simulink model "sowavedec2embd"  (R2012a)
settings: Solver=FixedStepDiscrete  StartTime=0.0  StopTime=inf  RelTol=1e-3
libraries: embdlinuxlib x2
settings Model: ExtModeTrigDuration=100  Creator=harashin  LastModifiedBy=Shogo
settings DataIOCC: LimitDataPoints=on  SaveFormat=Array  ReturnWorkspaceOutputs=off
settings OptimizationCC: ExpressionDepthLimit=2147483647  OptimizeModelRefInitCode=on  LifeSpan=1  SimCompilerOptimization=Off
settings DebuggingCC: UnderspecifiedInitializationDetection=Classic  MergeDetectMultiDrivingBlocksExec=none  FcnCallInpInsideContextMsg=Enable All  FrameProcessingCompatibilityMsg=warning  StateNameClashWarn=warning  StrictBusMsg=Warning  SFUnexpectedBacktrackingDiag=warning  SFNoUnconditionalDefaultTransitionDiag=warning
settings HardwareCC: ProdBitPerPointer=32  ProdLargestAtomicInteger=Long  ProdLargestAtomicFloat=Double  ProdIntDivRoundTo=Undefined  ProdWordSize=32  ProdHWDeviceType=ARM Compatible->ARM Cortex
settings ModelReferenceCC: PropagateSignalLabelsOutOfModel=off
settings SFSimCC: SimUseLocalCustomCode=off
settings RTWCC: SystemTargetFile=realtime.tlc  GenerateMakefile=off  TemplateMakefile=realtime.tmf  Description=Real-Time Toolbox  RTWVerbose=off  ProcessScript=realtime_make_rtw_hook  RTWUseLocalCustomCode=off  RTWCompilerOptimization=Off
settings CodeAppCC: CustomSymbolStrType=$N$R$M
settings STFCustomTargetCC: TargetLibSuffix=.a  CodeReplacementLibrary=ANSI_C  GenerateSampleERTMain=on  ERTCustomFileBanners=on  SupportNonInlinedSFcns=off  SupportVariableSizeSignals=on  GRTInterface=off  SystemTargetFile=realtime.tlc
settings ERTTargetCC: CodeReplacementLibrary=ANSI_C  MultiwordLength=2048  GenerateSampleERTMain=on  ParMdlRefBuildCompliant=off  CompOptLevelCompliant=off  ConcurrentExecutionCompliant=off  CombineOutputUpdateFcns=off  ERTFirstTimeCompliant=off  SupportContinuousTime=on  SupportVariableSizeSignals=on  ModelStepFunctionPrototypeControlCompliant=off  CPPClassGenCompliant=off  ExtModeMexArgs='192.168.111.22' 0 17725  InlinedParameterPlacement=NonHierarchical  ERTSrcFileBannerTemplate=realtime_code_template.cgt  ERTHdrFileBannerTemplate=realtime_code_template.cgt  ERTDataSrcFileTemplate=realtime_code_template.cgt  ERTDataHdrFileTemplate=realtime_code_template.cgt  ERTCustomFileTemplate=realtime_file_process.tlc  ConvertIfToSwitch=off  SuppressUnreachableDefaultCases=off  MemSecPackage=Simulink

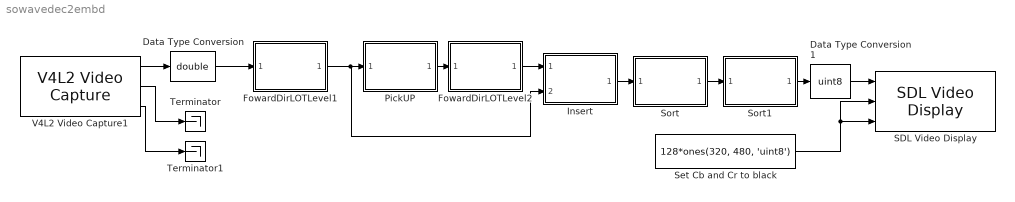
== system sowavedec2embd ==
  Data Type Conversion : DataTypeConversion  OutDataTypeStr=double
  Data Type Conversion1 : DataTypeConversion  OutDataTypeStr=uint8  SaturateOnIntegerOverflow=on
  FowardDirLOTLevel1 : MATLAB Function  TreatAsAtomicUnit=on
      settings: PermitHierarchicalResolution=ParametersOnly
  FowardDirLOTLevel2 : MATLAB Function  TreatAsAtomicUnit=on
      settings: PermitHierarchicalResolution=ParametersOnly
  Insert : MATLAB Function  TreatAsAtomicUnit=on
      settings: PermitHierarchicalResolution=ParametersOnly
  PickUP : MATLAB Function  TreatAsAtomicUnit=on
      settings: PermitHierarchicalResolution=ParametersOnly
  SDL Video Display : embdlinuxlib/SDL Video Display  pixelFormat=YCbCr 4:2:2  pixelOrder=Planar  rowMajor=on  blockPlatform=BeagleBoard
  Set Cb and Cr to black : Constant  Value=128*ones(320, 480, 'uint8')
  Sort : MATLAB Function  TreatAsAtomicUnit=on
      settings: PermitHierarchicalResolution=ParametersOnly
  Sort1 : MATLAB Function  TreatAsAtomicUnit=on
      settings: PermitHierarchicalResolution=ParametersOnly
  Terminator : Terminator
  Terminator1 : Terminator
  V4L2 Video Capture1 : embdlinuxlib/V4L2 Video Capture  m_devName='/dev/video0'  roi=[0, 0, 640, 480]  imSizeSelection=640x480  imSize=[640, 480]  pixelFormat=YCbCr 4:2:2  pixelOrder=Planar  sampleTime=1/10  simOutput=Colorbars  blockPlatform=BeagleBoard
  wires:
  Set Cb and Cr to black/1 -> SDL Video Display/3, SDL Video Display/2
  V4L2 Video Capture1/2 -> Terminator/1
  V4L2 Video Capture1/3 -> Terminator1/1
  V4L2 Video Capture1/1 -> Data Type Conversion/1
  Data Type Conversion1/1 -> SDL Video Display/1
  FowardDirLOTLevel1/1(coefActual) -> Insert/2(srcImg2), PickUP/1(srcImg)
  Data Type Conversion/1 -> FowardDirLOTLevel1/1(srcImg)
  PickUP/1(coefActual) -> FowardDirLOTLevel2/1(srcImg)
  FowardDirLOTLevel2/1(coefActual) -> Insert/1(srcImg1)
  Insert/1(coefActual) -> Sort/1(srcImg)
  Sort/1(coefActual) -> Sort1/1(srcImg)
  Sort1/1(coefActual) -> Data Type Conversion1/1

== matlab function sowavedec2embd/PickUP ==
  data: srcImg input; coefActual output
function coefActual = fcn(srcImg) %#codegen
%[ coefActual ] = coefPickUp(srcImg);
persistent hp;

if isempty(hp)
    
    % Instantiation
    hp = PickUp();
end

% Actual values
coefActual = step(hp,srcImg);

== matlab function sowavedec2embd/FowardDirLOTLevel1 ==
  data: srcImg input; coefActual output
function coefActual = fcn(srcImg) %#codegen 
%[ coefActual ] = forwardDirLot(srcImg);
persistent hf;
if isempty(hf)
    % Instantiation
    hf = ForwardDirLotEmb();
end
% Actual values
coefActual = step(hf,srcImg);

== matlab function sowavedec2embd/FowardDirLOTLevel2 ==
  data: srcImg input; coefActual output
function coefActual = fcn(srcImg) %#codegen
%[ coefActual ] = forwardDirLot(srcImg);
persistent hf;
if isempty(hf)
    % Instantiation
    hf = ForwardDirLotEmb();
end
% Actual values
coefActual = step(hf,srcImg);

== matlab function sowavedec2embd/Insert ==
  data: srcImg1 input; coefActual output; srcImg2 input
function coefActual = fcn(srcImg1,srcImg2) %#codegen
%[ coefActual ] = coefInsert(srcImg1,srcImg2);
persistent hi;

if isempty(hi)
    % Instantiation
    hi = Insert();
end

% Actual values
coefActual = step(hi,srcImg1,srcImg2);

== matlab function sowavedec2embd/Sort ==
  data: srcImg input; coefActual output
function coefActual = fcn(srcImg) %#codegen
%coefActual = SortCall(srcImg);
persistent hs;
if isempty(hs)
    % Instantiation
    hs = Sort();
end
% Actual values
coefActual = step(hs,srcImg);

== matlab function sowavedec2embd/Sort1 ==
  data: srcImg input; coefActual output
function coefActual = fcn(srcImg) %#codegen
persistent hs;
if isempty(hs)
    % Instantiation
    hs = Sort();
end

[nRows, nCols] = size(srcImg);
coefLL = srcImg(1:nRows/2,1:nCols/2);
%afterSortLL = SortCall(coefLL);
afterSortLL = step(hs,coefLL);

srcImg(1:nRows/2,1:nCols/2) = afterSortLL;

srcImg2 = zeros(nRows,nCols);
srcImg2(1:nRows/4,1:nCols/4) = srcImg(1:nRows/4,1:nCols/4)*0.3;
srcImg2(nRows/4+1:nRows/2,1:nCols/4) = srcImg(nRows/4+1:nRows/2,1:nCols/4)*4;
srcImg2(1:nRows/4,nCols/4+1:nCols/2) = srcImg(1:nRows/4,nCols/4+1:nCols/2)*4;
srcImg2(nRows/4+1:nRows/2,nCols/4+1:nCols/2) = ...
    srcImg(nRows/4+1:nRows/2,nCols/4+1:nCols/2)*4;
srcImg2(nRows/2+1:nRows,1:nCols/2) = srcImg(nRows/2+1:nRows,1:nCols/2)*6;
srcImg2(1:nRows/2,nCols/2+1:nCols) = srcImg(1:nRows/2,nCols/2+1:nCols)*6;
srcImg2(nRows/2+1:nRows,nCols/2+1:nCols) = ...
    srcImg(nRows/2+1:nRows,nCols/2+1:nCols)*6;


coefActual = srcImg2;
